simulink subsystem "ring_oscillator_stage"  (R2020b)
settings: Solver=VariableStepAuto  StartTime=0.0  StopTime=10.0  RelTol=1e-3
model mask{tau=1, alpha=1, beta=1, x0=1}
  mask prompts: tau "\tau"; alpha "\alpha"; beta "\beta"
values from neighbouring files (symbols this model uses):
  alpha = 1    [MECH6313_HW6_pblm3.m]
  beta = mu/alpha    [MECH6313_HW6_pblm3.m]
  tau = 1    [MECH6313_HW6_pblm3.m]
  x0 = 1    [MECH6313_HW6_pblm3.m]
settings Model: Creator=Jonas  LastModifiedBy=Jonas

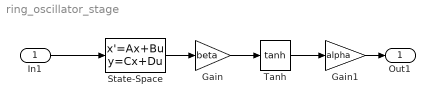
== system ring_oscillator_stage ==
  In1 : Inport
  Gain : Gain  Gain=beta
  Gain1 : Gain  Gain=alpha
  State-Space : StateSpace  A=-1/tau  B=1/tau  D=0  InitialCondition=x0
  Tanh : Trigonometry  Operator=tanh
  Out1 : Outport
  wires:
  In1/1 -> State-Space/1
  State-Space/1 -> Gain/1
  Gain/1 -> Tanh/1
  Gain1/1 -> Out1/1
  Tanh/1 -> Gain1/1
